simulink model "simTopLevel"  (R2016b)
settings: Solver=ode15s  StartTime=0.0  StopTime=2  RelTol=1e-3  EnableMultiTasking=on
InitFcn:
  | % minitaurParameters
model workspace (MAT data in the model file):
  MCOS : class17 (value not decoded)
  MCOS : class17 (value not decoded)
  MCOS : class17 (value not decoded)
  MCOS : class17 (value not decoded)
values from neighbouring files (symbols this model uses):
  controlParams = Simulink.Parameter(controlParams)    [minitaurParameters.m]
  envParams = Simulink.Parameter(envParams)    [minitaurParameters.m]
  IC = Simulink.Parameter(IC)    [minitaurParameters.m]
  minitaurParams = Simulink.Parameter(minitaurParams)    [minitaurParameters.m]
undefined symbols (not defined in the file or in its folder): Axis, Fn, ForeRearLag, Period, tau0, tau1, X, Y, Z
libraries: sm_lib x464, fl_lib x132, nesl_utility x41, Contact_Forces_Lib x28, simulink x13, simulink_extras x1
(part 11 of 13)

== system simTopLevel/GR Minitaur/minitaur_leg_linkages_III/Joint Friction Model1/Full ==
  Ideal Force Sensor : fl_lib/Mechanical/Mechanical Sensors/Ideal Force Sensor
  Ideal Translational Velocity Source : fl_lib/Mechanical/Mechanical Sources/Ideal Translational Velocity Source
  Joint Diameter : fl_lib/Physical Signals/Functions/PS Gain  gain=2*leg_joint_radius
  Joint Radius : fl_lib/Physical Signals/Functions/PS Gain  gain=leg_joint_radius
  Mechanical Translational Reference : fl_lib/Mechanical/Translational Elements/Mechanical Translational Reference
  Mechanical Translational Reference1 : fl_lib/Mechanical/Translational Elements/Mechanical Translational Reference
  PS Terminator : fl_lib/Physical Signals/Sinks/PS Terminator
  Translational Friction : fl_lib/Mechanical/Translational Elements/Translational Friction  brkwy_frc=mu_brk*Fn N  Col_frc=mu_k*Fn N  visc_coef=fric_visc_coeff N/(m/s)  trans_coef=trans_coeff s/m  vel_thr=linear_region_thresh m/s  v_specify=off  v_priority=None  v=0 m/s  f_specify=off  f_priority=None  f=0 N
  Joint Angular Velocity : PMIOPort  Port=1  Side=Left
  Joint Force : PMIOPort  Port=2  Side=Left
  Friction Torque : PMIOPort  Port=3  Side=Right
  connections:
  Mechanical Translational Reference/LConn1 -- Ideal Force Sensor/RConn1
  Translational Friction/LConn1 -- Ideal Force Sensor/LConn1
  Translational Friction/RConn1 -- Ideal Translational Velocity Source/LConn1
  Ideal Force Sensor/RConn2 -- Joint Diameter/LConn1
  Joint Diameter/RConn1 -- Friction Torque/RConn1
  Mechanical Translational Reference1/LConn1 -- Ideal Translational Velocity Source/RConn2
  Joint Force/RConn1 -- PS Terminator/LConn1
  Joint Radius/LConn1 -- Joint Angular Velocity/RConn1
  Joint Radius/RConn1 -- Ideal Translational Velocity Source/RConn1

== system simTopLevel/GR Minitaur/minitaur_leg_linkages_III/Joint Friction Model1/Stick-Slip ==
  Joint Diameter : fl_lib/Physical Signals/Functions/PS Gain  gain=2*leg_joint_radius
  Joint Radius : fl_lib/Physical Signals/Functions/PS Gain  gain=leg_joint_radius
  PS Add : fl_lib/Physical Signals/Functions/PS Add
  Stick-Slip Friction X : Contact_Forces_Lib/Friction Utilities/Stick-Slip Friction 1D  fn_axis=X-Axis  mu_kinetic=mu_k/2  mu_static=mu_s/2  vel_th=linear_region_thresh  filt_const=1/(2*pi*fric_bandwidth)
  Stick-Slip Friction Y : Contact_Forces_Lib/Friction Utilities/Stick-Slip Friction 1D  fn_axis=Y-Axis  mu_kinetic=mu_k/2  mu_static=mu_s/2  vel_th=linear_region_thresh  filt_const=1/(2*pi*fric_bandwidth)
  Joint Angular Velocity : PMIOPort  Port=1  Side=Left
  Joint Force : PMIOPort  Port=2  Side=Left
  Friction Torque : PMIOPort  Port=3  Side=Right
  connections:
  Joint Radius/RConn1 -- Stick-Slip Friction X/LConn2 -- Stick-Slip Friction Y/LConn2
  Joint Force/RConn1 -- Stick-Slip Friction X/LConn1 -- Stick-Slip Friction Y/LConn1
  Stick-Slip Friction Y/RConn1 -- PS Add/LConn2
  Stick-Slip Friction X/RConn1 -- PS Add/LConn1
  Joint Diameter/LConn1 -- PS Add/RConn1
  Joint Diameter/RConn1 -- Friction Torque/RConn1
  Joint Radius/LConn1 -- Joint Angular Velocity/RConn1

== system simTopLevel/GR Minitaur/minitaur_leg_linkages_III/Joint Friction Model2/Full ==
  Ideal Force Sensor : fl_lib/Mechanical/Mechanical Sensors/Ideal Force Sensor
  Ideal Translational Velocity Source : fl_lib/Mechanical/Mechanical Sources/Ideal Translational Velocity Source
  Joint Diameter : fl_lib/Physical Signals/Functions/PS Gain  gain=2*leg_joint_radius
  Joint Radius : fl_lib/Physical Signals/Functions/PS Gain  gain=leg_joint_radius
  Mechanical Translational Reference : fl_lib/Mechanical/Translational Elements/Mechanical Translational Reference
  Mechanical Translational Reference1 : fl_lib/Mechanical/Translational Elements/Mechanical Translational Reference
  PS Terminator : fl_lib/Physical Signals/Sinks/PS Terminator
  Translational Friction : fl_lib/Mechanical/Translational Elements/Translational Friction  brkwy_frc=mu_brk*Fn N  Col_frc=mu_k*Fn N  visc_coef=fric_visc_coeff N/(m/s)  trans_coef=trans_coeff s/m  vel_thr=linear_region_thresh m/s  v_specify=off  v_priority=None  v=0 m/s  f_specify=off  f_priority=None  f=0 N
  Joint Angular Velocity : PMIOPort  Port=1  Side=Left
  Joint Force : PMIOPort  Port=2  Side=Left
  Friction Torque : PMIOPort  Port=3  Side=Right
  connections:
  Mechanical Translational Reference/LConn1 -- Ideal Force Sensor/RConn1
  Translational Friction/LConn1 -- Ideal Force Sensor/LConn1
  Translational Friction/RConn1 -- Ideal Translational Velocity Source/LConn1
  Ideal Force Sensor/RConn2 -- Joint Diameter/LConn1
  Joint Diameter/RConn1 -- Friction Torque/RConn1
  Mechanical Translational Reference1/LConn1 -- Ideal Translational Velocity Source/RConn2
  Joint Force/RConn1 -- PS Terminator/LConn1
  Joint Radius/LConn1 -- Joint Angular Velocity/RConn1
  Joint Radius/RConn1 -- Ideal Translational Velocity Source/RConn1

== system simTopLevel/GR Minitaur/minitaur_leg_linkages_III/Joint Friction Model2/Stick-Slip ==
  Joint Diameter : fl_lib/Physical Signals/Functions/PS Gain  gain=2*leg_joint_radius
  Joint Radius : fl_lib/Physical Signals/Functions/PS Gain  gain=leg_joint_radius
  PS Add : fl_lib/Physical Signals/Functions/PS Add
  Stick-Slip Friction X : Contact_Forces_Lib/Friction Utilities/Stick-Slip Friction 1D  fn_axis=X-Axis  mu_kinetic=mu_k/2  mu_static=mu_s/2  vel_th=linear_region_thresh  filt_const=1/(2*pi*fric_bandwidth)
  Stick-Slip Friction Y : Contact_Forces_Lib/Friction Utilities/Stick-Slip Friction 1D  fn_axis=Y-Axis  mu_kinetic=mu_k/2  mu_static=mu_s/2  vel_th=linear_region_thresh  filt_const=1/(2*pi*fric_bandwidth)
  Joint Angular Velocity : PMIOPort  Port=1  Side=Left
  Joint Force : PMIOPort  Port=2  Side=Left
  Friction Torque : PMIOPort  Port=3  Side=Right
  connections:
  Joint Radius/RConn1 -- Stick-Slip Friction X/LConn2 -- Stick-Slip Friction Y/LConn2
  Joint Force/RConn1 -- Stick-Slip Friction X/LConn1 -- Stick-Slip Friction Y/LConn1
  Stick-Slip Friction Y/RConn1 -- PS Add/LConn2
  Stick-Slip Friction X/RConn1 -- PS Add/LConn1
  Joint Diameter/LConn1 -- PS Add/RConn1
  Joint Diameter/RConn1 -- Friction Torque/RConn1
  Joint Radius/LConn1 -- Joint Angular Velocity/RConn1

== system simTopLevel/GR Minitaur/minitaur_leg_linkages_IV/Joint Friction Model/Full ==
  Ideal Force Sensor : fl_lib/Mechanical/Mechanical Sensors/Ideal Force Sensor
  Ideal Translational Velocity Source : fl_lib/Mechanical/Mechanical Sources/Ideal Translational Velocity Source
  Joint Diameter : fl_lib/Physical Signals/Functions/PS Gain  gain=2*leg_joint_radius
  Joint Radius : fl_lib/Physical Signals/Functions/PS Gain  gain=leg_joint_radius
  Mechanical Translational Reference : fl_lib/Mechanical/Translational Elements/Mechanical Translational Reference
  Mechanical Translational Reference1 : fl_lib/Mechanical/Translational Elements/Mechanical Translational Reference
  PS Terminator : fl_lib/Physical Signals/Sinks/PS Terminator
  Translational Friction : fl_lib/Mechanical/Translational Elements/Translational Friction  brkwy_frc=mu_brk*Fn N  Col_frc=mu_k*Fn N  visc_coef=fric_visc_coeff N/(m/s)  trans_coef=trans_coeff s/m  vel_thr=linear_region_thresh m/s  v_specify=off  v_priority=None  v=0 m/s  f_specify=off  f_priority=None  f=0 N
  Joint Angular Velocity : PMIOPort  Port=1  Side=Left
  Joint Force : PMIOPort  Port=2  Side=Left
  Friction Torque : PMIOPort  Port=3  Side=Right
  connections:
  Mechanical Translational Reference/LConn1 -- Ideal Force Sensor/RConn1
  Translational Friction/LConn1 -- Ideal Force Sensor/LConn1
  Translational Friction/RConn1 -- Ideal Translational Velocity Source/LConn1
  Ideal Force Sensor/RConn2 -- Joint Diameter/LConn1
  Joint Diameter/RConn1 -- Friction Torque/RConn1
  Mechanical Translational Reference1/LConn1 -- Ideal Translational Velocity Source/RConn2
  Joint Force/RConn1 -- PS Terminator/LConn1
  Joint Radius/LConn1 -- Joint Angular Velocity/RConn1
  Joint Radius/RConn1 -- Ideal Translational Velocity Source/RConn1

== system simTopLevel/GR Minitaur/minitaur_leg_linkages_IV/Joint Friction Model/Stick-Slip ==
  Joint Diameter : fl_lib/Physical Signals/Functions/PS Gain  gain=2*leg_joint_radius
  Joint Radius : fl_lib/Physical Signals/Functions/PS Gain  gain=leg_joint_radius
  PS Add : fl_lib/Physical Signals/Functions/PS Add
  Stick-Slip Friction X : Contact_Forces_Lib/Friction Utilities/Stick-Slip Friction 1D  fn_axis=X-Axis  mu_kinetic=mu_k/2  mu_static=mu_s/2  vel_th=linear_region_thresh  filt_const=1/(2*pi*fric_bandwidth)
  Stick-Slip Friction Y : Contact_Forces_Lib/Friction Utilities/Stick-Slip Friction 1D  fn_axis=Y-Axis  mu_kinetic=mu_k/2  mu_static=mu_s/2  vel_th=linear_region_thresh  filt_const=1/(2*pi*fric_bandwidth)
  Joint Angular Velocity : PMIOPort  Port=1  Side=Left
  Joint Force : PMIOPort  Port=2  Side=Left
  Friction Torque : PMIOPort  Port=3  Side=Right
  connections:
  Joint Radius/RConn1 -- Stick-Slip Friction X/LConn2 -- Stick-Slip Friction Y/LConn2
  Joint Force/RConn1 -- Stick-Slip Friction X/LConn1 -- Stick-Slip Friction Y/LConn1
  Stick-Slip Friction Y/RConn1 -- PS Add/LConn2
  Stick-Slip Friction X/RConn1 -- PS Add/LConn1
  Joint Diameter/LConn1 -- PS Add/RConn1
  Joint Diameter/RConn1 -- Friction Torque/RConn1
  Joint Radius/LConn1 -- Joint Angular Velocity/RConn1

== system simTopLevel/GR Minitaur/minitaur_leg_linkages_IV/Joint Friction Model1/Full ==
  Ideal Force Sensor : fl_lib/Mechanical/Mechanical Sensors/Ideal Force Sensor
  Ideal Translational Velocity Source : fl_lib/Mechanical/Mechanical Sources/Ideal Translational Velocity Source
  Joint Diameter : fl_lib/Physical Signals/Functions/PS Gain  gain=2*leg_joint_radius
  Joint Radius : fl_lib/Physical Signals/Functions/PS Gain  gain=leg_joint_radius
  Mechanical Translational Reference : fl_lib/Mechanical/Translational Elements/Mechanical Translational Reference
  Mechanical Translational Reference1 : fl_lib/Mechanical/Translational Elements/Mechanical Translational Reference
  PS Terminator : fl_lib/Physical Signals/Sinks/PS Terminator
  Translational Friction : fl_lib/Mechanical/Translational Elements/Translational Friction  brkwy_frc=mu_brk*Fn N  Col_frc=mu_k*Fn N  visc_coef=fric_visc_coeff N/(m/s)  trans_coef=trans_coeff s/m  vel_thr=linear_region_thresh m/s  v_specify=off  v_priority=None  v=0 m/s  f_specify=off  f_priority=None  f=0 N
  Joint Angular Velocity : PMIOPort  Port=1  Side=Left
  Joint Force : PMIOPort  Port=2  Side=Left
  Friction Torque : PMIOPort  Port=3  Side=Right
  connections:
  Mechanical Translational Reference/LConn1 -- Ideal Force Sensor/RConn1
  Translational Friction/LConn1 -- Ideal Force Sensor/LConn1
  Translational Friction/RConn1 -- Ideal Translational Velocity Source/LConn1
  Ideal Force Sensor/RConn2 -- Joint Diameter/LConn1
  Joint Diameter/RConn1 -- Friction Torque/RConn1
  Mechanical Translational Reference1/LConn1 -- Ideal Translational Velocity Source/RConn2
  Joint Force/RConn1 -- PS Terminator/LConn1
  Joint Radius/LConn1 -- Joint Angular Velocity/RConn1
  Joint Radius/RConn1 -- Ideal Translational Velocity Source/RConn1

== system simTopLevel/GR Minitaur/minitaur_leg_linkages_IV/Joint Friction Model1/Stick-Slip ==
  Joint Diameter : fl_lib/Physical Signals/Functions/PS Gain  gain=2*leg_joint_radius
  Joint Radius : fl_lib/Physical Signals/Functions/PS Gain  gain=leg_joint_radius
  PS Add : fl_lib/Physical Signals/Functions/PS Add
  Stick-Slip Friction X : Contact_Forces_Lib/Friction Utilities/Stick-Slip Friction 1D  fn_axis=X-Axis  mu_kinetic=mu_k/2  mu_static=mu_s/2  vel_th=linear_region_thresh  filt_const=1/(2*pi*fric_bandwidth)
  Stick-Slip Friction Y : Contact_Forces_Lib/Friction Utilities/Stick-Slip Friction 1D  fn_axis=Y-Axis  mu_kinetic=mu_k/2  mu_static=mu_s/2  vel_th=linear_region_thresh  filt_const=1/(2*pi*fric_bandwidth)
  Joint Angular Velocity : PMIOPort  Port=1  Side=Left
  Joint Force : PMIOPort  Port=2  Side=Left
  Friction Torque : PMIOPort  Port=3  Side=Right
  connections:
  Joint Radius/RConn1 -- Stick-Slip Friction X/LConn2 -- Stick-Slip Friction Y/LConn2
  Joint Force/RConn1 -- Stick-Slip Friction X/LConn1 -- Stick-Slip Friction Y/LConn1
  Stick-Slip Friction Y/RConn1 -- PS Add/LConn2
  Stick-Slip Friction X/RConn1 -- PS Add/LConn1
  Joint Diameter/LConn1 -- PS Add/RConn1
  Joint Diameter/RConn1 -- Friction Torque/RConn1
  Joint Radius/LConn1 -- Joint Angular Velocity/RConn1

== system simTopLevel/GR Minitaur/minitaur_leg_linkages_IV/Joint Friction Model2/Full ==
  Ideal Force Sensor : fl_lib/Mechanical/Mechanical Sensors/Ideal Force Sensor
  Ideal Translational Velocity Source : fl_lib/Mechanical/Mechanical Sources/Ideal Translational Velocity Source
  Joint Diameter : fl_lib/Physical Signals/Functions/PS Gain  gain=2*leg_joint_radius
  Joint Radius : fl_lib/Physical Signals/Functions/PS Gain  gain=leg_joint_radius
  Mechanical Translational Reference : fl_lib/Mechanical/Translational Elements/Mechanical Translational Reference
  Mechanical Translational Reference1 : fl_lib/Mechanical/Translational Elements/Mechanical Translational Reference
  PS Terminator : fl_lib/Physical Signals/Sinks/PS Terminator
  Translational Friction : fl_lib/Mechanical/Translational Elements/Translational Friction  brkwy_frc=mu_brk*Fn N  Col_frc=mu_k*Fn N  visc_coef=fric_visc_coeff N/(m/s)  trans_coef=trans_coeff s/m  vel_thr=linear_region_thresh m/s  v_specify=off  v_priority=None  v=0 m/s  f_specify=off  f_priority=None  f=0 N
  Joint Angular Velocity : PMIOPort  Port=1  Side=Left
  Joint Force : PMIOPort  Port=2  Side=Left
  Friction Torque : PMIOPort  Port=3  Side=Right
  connections:
  Mechanical Translational Reference/LConn1 -- Ideal Force Sensor/RConn1
  Translational Friction/LConn1 -- Ideal Force Sensor/LConn1
  Translational Friction/RConn1 -- Ideal Translational Velocity Source/LConn1
  Ideal Force Sensor/RConn2 -- Joint Diameter/LConn1
  Joint Diameter/RConn1 -- Friction Torque/RConn1
  Mechanical Translational Reference1/LConn1 -- Ideal Translational Velocity Source/RConn2
  Joint Force/RConn1 -- PS Terminator/LConn1
  Joint Radius/LConn1 -- Joint Angular Velocity/RConn1
  Joint Radius/RConn1 -- Ideal Translational Velocity Source/RConn1

== system simTopLevel/GR Minitaur/minitaur_leg_linkages_IV/Joint Friction Model2/Stick-Slip ==
  Joint Diameter : fl_lib/Physical Signals/Functions/PS Gain  gain=2*leg_joint_radius
  Joint Radius : fl_lib/Physical Signals/Functions/PS Gain  gain=leg_joint_radius
  PS Add : fl_lib/Physical Signals/Functions/PS Add
  Stick-Slip Friction X : Contact_Forces_Lib/Friction Utilities/Stick-Slip Friction 1D  fn_axis=X-Axis  mu_kinetic=mu_k/2  mu_static=mu_s/2  vel_th=linear_region_thresh  filt_const=1/(2*pi*fric_bandwidth)
  Stick-Slip Friction Y : Contact_Forces_Lib/Friction Utilities/Stick-Slip Friction 1D  fn_axis=Y-Axis  mu_kinetic=mu_k/2  mu_static=mu_s/2  vel_th=linear_region_thresh  filt_const=1/(2*pi*fric_bandwidth)
  Joint Angular Velocity : PMIOPort  Port=1  Side=Left
  Joint Force : PMIOPort  Port=2  Side=Left
  Friction Torque : PMIOPort  Port=3  Side=Right
  connections:
  Joint Radius/RConn1 -- Stick-Slip Friction X/LConn2 -- Stick-Slip Friction Y/LConn2
  Joint Force/RConn1 -- Stick-Slip Friction X/LConn1 -- Stick-Slip Friction Y/LConn1
  Stick-Slip Friction Y/RConn1 -- PS Add/LConn2
  Stick-Slip Friction X/RConn1 -- PS Add/LConn1
  Joint Diameter/LConn1 -- PS Add/RConn1
  Joint Diameter/RConn1 -- Friction Torque/RConn1
  Joint Radius/LConn1 -- Joint Angular Velocity/RConn1

== system simTopLevel/GR Minitaur/minitaur_motor_module_IA/DYS_BLDC_86x10_BE8108_12/BLDC Model ==
  Desired Torque  [Nm] : Inport
  Velocity [rad/s] : Inport  Port=2
  Constant : Constant  Value=torque_sat
  Constant1 : Constant  Value=-torque_sat
  Gain : Gain  Gain=1/kt
  Gain1 : Gain  Gain=r
  Math Function : Math  Operator=square  SaturateOnIntegerOverflow=on
  Saturation Dynamic : simulink/Discontinuities/Saturation Dynamic  OutMin=[]  OutMax=[]  OutDataTypeStr=Inherit: Same as second input  OutDataType=fixdt(1, 16)  OutScaling=2^-10  DoSatur=off
  Terminator : Terminator
  Transfer Fcn : TransferFcn  Denominator=[timeconst 1]
  Torque [N*m] : Outport
  Ploss [W] : Outport  Port=2
  wires:
  Desired Torque  [Nm]/1 -> Transfer Fcn/1
  Math Function/1 -> Gain1/1
  Gain/1 -> Math Function/1
  Gain1/1 -> Ploss [W]/1
  Velocity [rad/s]/1 -> Terminator/1
  Transfer Fcn/1 -> Saturation Dynamic/2
  Saturation Dynamic/1 -> Gain/1, Torque [N*m]/1
  Constant/1 -> Saturation Dynamic/1
  Constant1/1 -> Saturation Dynamic/3

== system simTopLevel/GR Minitaur/minitaur_motor_module_IA/DYS_BLDC_86x10_BE8108_12/DYS_BLDC_86x10_BE8108_12_rotor_1_RIGID ==
  ReferenceFrame : sm_lib/Frames and Transforms/Reference Frame
  Solid : sm_lib/Body Elements/Solid  InertiaType=Custom  Mass=minitaurParams.Solid(7).mass  MassUnits=kg  CenterOfMass=minitaurParams.Solid(7).CoM  CenterOfMassUnits=mm  MomentsOfInertia=minitaurParams.Solid(7).MoI  MomentsOfInertiaUnits=kg*mm^2  ProductsOfInertia=minitaurParams.Solid(7).PoI  ProductsOfInertiaUnits=kg*mm^2  DensityBased=on  Density=1000  DensityUnits=kg/(m^3)  DoExposeReferenceFrame=on  SerializedFrames=<Frames/>  GraphicType=FromGeometry  MarkerShape=Sphere  MarkerSize=10  GraphicVisPropType=SimpleVisualProperties  GraphicDiffuseColor=minitaurParams.Solid(7).color  GraphicSpecularColor=[0.5 0.5 0.5 1.0]  GraphicAmbientColor=[0.15 0.15 0.15 1.0]  GraphicEmissiveColor=[0.0 0.0 0.0 1.0]  GraphicShininess=75  GraphicOpacity=minitaurParams.Solid(7).opacity  GeometryShape=FromFile  RectangleSize=[1 1]  RectangleSizeUnits=m  BrickDimensions=[1 1 1]  BrickDimensionUnits=m  CylinderRadius=1  CylinderRadiusUnits=m  CylinderLength=1  CylinderLengthUnits=m  SphereRadius=1  SphereRadiusUnits=m  EllipsoidRadii=[1 1 1]  EllipsoidRadiiUnits=m  ExtrusionCrossSection=[1 1; -1 1; -1 -1; 1 -1]  ExtrusionCrossSectionUnits=m  ExtrusionLength=1  ExtrusionLengthUnits=m  PolygonNumSides=3  PolygonOuterRadius=1  PolygonOuterRadiusUnits=m  ExtGeomFileType=STEP  ExtGeomFileName=model/DYS-BLDC-86x10-BE8108-12-rotor_Default_sldprt.STEP  ExtGeomFileUnits=m  RevolutionCrossSection=[1 1; 1 -1; 2 -1; 2 1]  RevolutionCrossSectionUnits=m  RevolutionExtent=Full  RevolutionAngle=180  RevolutionAngleUnits=deg
  Transform : sm_lib/Frames and Transforms/Rigid Transform  TranslationMethod=Cartesian  TranslationStandardOffset=0  TranslationLengthUnit=mm  TranslationStandardAxis=+Z  TranslationCartesianOffset=minitaurParams.RigidTransform(20).translation  TranslationROffset=0  TranslationROffsetUnits=m  TranslationZOffset=0  TranslationZOffsetUnits=m  TranslationThetaOffset=0  TranslationThetaOffsetUnits=deg  RotationMethod=ArbitraryAxis  RotationAngleUnits=rad  RotationStandardAxis=+Z  RotationAngle=minitaurParams.RigidTransform(20).angle  RotationArbitraryAxis=minitaurParams.RigidTransform(20).axis  FollAlignAxisA=+X  BaseAlignAxisA=+Y  FollAlignAxisB=+Y  BaseAlignAxisB=+Z  RotationSequenceAxes=FollowerAxes  RotationSequence=XYX  RotationSequenceAngles=[0 0 0]  RotationSequenceAnglesUnits=deg  RotationMatrix=[1 0 0; 0 1 0; 0 0 1]
  Transform1 : sm_lib/Frames and Transforms/Rigid Transform  TranslationMethod=Cartesian  TranslationStandardOffset=0  TranslationLengthUnit=mm  TranslationStandardAxis=+Z  TranslationCartesianOffset=minitaurParams.RigidTransform(48).translation  TranslationROffset=0  TranslationROffsetUnits=m  TranslationZOffset=0  TranslationZOffsetUnits=m  TranslationThetaOffset=0  TranslationThetaOffsetUnits=deg  RotationMethod=ArbitraryAxis  RotationAngleUnits=rad  RotationStandardAxis=+Z  RotationAngle=minitaurParams.RigidTransform(48).angle  RotationArbitraryAxis=minitaurParams.RigidTransform(48).axis  FollAlignAxisA=+X  BaseAlignAxisA=+Y  FollAlignAxisB=+Y  BaseAlignAxisB=+Z  RotationSequenceAxes=FollowerAxes  RotationSequence=XYX  RotationSequenceAngles=[0 0 0]  RotationSequenceAnglesUnits=deg  RotationMatrix=[1 0 0; 0 1 0; 0 0 1]
  F1 : PMIOPort  Port=1  Side=Left
  F : PMIOPort  Port=2  Side=Left
  connections:
  ReferenceFrame/RConn1 -- Solid/RConn1 -- Transform/LConn1 -- Transform1/LConn1
  Transform/RConn1 -- F/RConn1
  Transform1/RConn1 -- F1/RConn1

== system simTopLevel/GR Minitaur/minitaur_motor_module_IA/DYS_BLDC_86x10_BE8108_12/DYS_BLDC_86x10_BE8108_12_stator_1_RIGID ==
  ReferenceFrame : sm_lib/Frames and Transforms/Reference Frame
  Solid : sm_lib/Body Elements/Solid  InertiaType=Custom  Mass=minitaurParams.Solid(6).mass  MassUnits=kg  CenterOfMass=minitaurParams.Solid(6).CoM  CenterOfMassUnits=mm  MomentsOfInertia=minitaurParams.Solid(6).MoI  MomentsOfInertiaUnits=kg*mm^2  ProductsOfInertia=minitaurParams.Solid(6).PoI  ProductsOfInertiaUnits=kg*mm^2  DensityBased=on  Density=1000  DensityUnits=kg/(m^3)  DoExposeReferenceFrame=on  SerializedFrames=<Frames/>  GraphicType=FromGeometry  MarkerShape=Sphere  MarkerSize=10  GraphicVisPropType=SimpleVisualProperties  GraphicDiffuseColor=minitaurParams.Solid(6).color  GraphicSpecularColor=[0.5 0.5 0.5 1.0]  GraphicAmbientColor=[0.15 0.15 0.15 1.0]  GraphicEmissiveColor=[0.0 0.0 0.0 1.0]  GraphicShininess=75  GraphicOpacity=minitaurParams.Solid(6).opacity  GeometryShape=FromFile  RectangleSize=[1 1]  RectangleSizeUnits=m  BrickDimensions=[1 1 1]  BrickDimensionUnits=m  CylinderRadius=1  CylinderRadiusUnits=m  CylinderLength=1  CylinderLengthUnits=m  SphereRadius=1  SphereRadiusUnits=m  EllipsoidRadii=[1 1 1]  EllipsoidRadiiUnits=m  ExtrusionCrossSection=[1 1; -1 1; -1 -1; 1 -1]  ExtrusionCrossSectionUnits=m  ExtrusionLength=1  ExtrusionLengthUnits=m  PolygonNumSides=3  PolygonOuterRadius=1  PolygonOuterRadiusUnits=m  ExtGeomFileType=STEP  ExtGeomFileName=model/DYS-BLDC-86x10-BE8108-12-stator_Default_sldprt.STEP  ExtGeomFileUnits=m  RevolutionCrossSection=[1 1; 1 -1; 2 -1; 2 1]  RevolutionCrossSectionUnits=m  RevolutionExtent=Full  RevolutionAngle=180  RevolutionAngleUnits=deg
  Transform : sm_lib/Frames and Transforms/Rigid Transform  TranslationMethod=Cartesian  TranslationStandardOffset=0  TranslationLengthUnit=mm  TranslationStandardAxis=+Z  TranslationCartesianOffset=minitaurParams.RigidTransform(17).translation  TranslationROffset=0  TranslationROffsetUnits=m  TranslationZOffset=0  TranslationZOffsetUnits=m  TranslationThetaOffset=0  TranslationThetaOffsetUnits=deg  RotationMethod=ArbitraryAxis  RotationAngleUnits=rad  RotationStandardAxis=+Z  RotationAngle=minitaurParams.RigidTransform(17).angle  RotationArbitraryAxis=minitaurParams.RigidTransform(17).axis  FollAlignAxisA=+X  BaseAlignAxisA=+Y  FollAlignAxisB=+Y  BaseAlignAxisB=+Z  RotationSequenceAxes=FollowerAxes  RotationSequence=XYX  RotationSequenceAngles=[0 0 0]  RotationSequenceAnglesUnits=deg  RotationMatrix=[1 0 0; 0 1 0; 0 0 1]
  Transform1 : sm_lib/Frames and Transforms/Rigid Transform  TranslationMethod=Cartesian  TranslationStandardOffset=0  TranslationLengthUnit=mm  TranslationStandardAxis=+Z  TranslationCartesianOffset=minitaurParams.RigidTransform(19).translation  TranslationROffset=0  TranslationROffsetUnits=m  TranslationZOffset=0  TranslationZOffsetUnits=m  TranslationThetaOffset=0  TranslationThetaOffsetUnits=deg  RotationMethod=ArbitraryAxis  RotationAngleUnits=rad  RotationStandardAxis=+Z  RotationAngle=minitaurParams.RigidTransform(19).angle  RotationArbitraryAxis=minitaurParams.RigidTransform(19).axis  FollAlignAxisA=+X  BaseAlignAxisA=+Y  FollAlignAxisB=+Y  BaseAlignAxisB=+Z  RotationSequenceAxes=FollowerAxes  RotationSequence=XYX  RotationSequenceAngles=[0 0 0]  RotationSequenceAnglesUnits=deg  RotationMatrix=[1 0 0; 0 1 0; 0 0 1]
  Transform2 : sm_lib/Frames and Transforms/Rigid Transform  TranslationMethod=Cartesian  TranslationStandardOffset=0  TranslationLengthUnit=mm  TranslationStandardAxis=+Z  TranslationCartesianOffset=minitaurParams.RigidTransform(26).translation  TranslationROffset=0  TranslationROffsetUnits=m  TranslationZOffset=0  TranslationZOffsetUnits=m  TranslationThetaOffset=0  TranslationThetaOffsetUnits=deg  RotationMethod=ArbitraryAxis  RotationAngleUnits=rad  RotationStandardAxis=+Z  RotationAngle=minitaurParams.RigidTransform(26).angle  RotationArbitraryAxis=minitaurParams.RigidTransform(26).axis  FollAlignAxisA=+X  BaseAlignAxisA=+Y  FollAlignAxisB=+Y  BaseAlignAxisB=+Z  RotationSequenceAxes=FollowerAxes  RotationSequence=XYX  RotationSequenceAngles=[0 0 0]  RotationSequenceAnglesUnits=deg  RotationMatrix=[1 0 0; 0 1 0; 0 0 1]
  Transform3 : sm_lib/Frames and Transforms/Rigid Transform  TranslationMethod=Cartesian  TranslationStandardOffset=0  TranslationLengthUnit=mm  TranslationStandardAxis=+Z  TranslationCartesianOffset=minitaurParams.RigidTransform(34).translation  TranslationROffset=0  TranslationROffsetUnits=m  TranslationZOffset=0  TranslationZOffsetUnits=m  TranslationThetaOffset=0  TranslationThetaOffsetUnits=deg  RotationMethod=ArbitraryAxis  RotationAngleUnits=rad  RotationStandardAxis=+Z  RotationAngle=minitaurParams.RigidTransform(34).angle  RotationArbitraryAxis=minitaurParams.RigidTransform(34).axis  FollAlignAxisA=+X  BaseAlignAxisA=+Y  FollAlignAxisB=+Y  BaseAlignAxisB=+Z  RotationSequenceAxes=FollowerAxes  RotationSequence=XYX  RotationSequenceAngles=[0 0 0]  RotationSequenceAnglesUnits=deg  RotationMatrix=[1 0 0; 0 1 0; 0 0 1]
  F2 : PMIOPort  Port=1  Side=Left
  F3 : PMIOPort  Port=2  Side=Left
  F : PMIOPort  Port=3  Side=Left
  F1 : PMIOPort  Port=4  Side=Right
  connections:
  Transform2/LConn1 -- Transform3/LConn1 -- ReferenceFrame/RConn1 -- Solid/RConn1 -- Transform/LConn1 -- Transform1/LConn1
  Transform/RConn1 -- F/RConn1
  Transform1/RConn1 -- F1/RConn1
  Transform2/RConn1 -- F2/RConn1
  Transform3/RConn1 -- F3/RConn1

== system simTopLevel/GR Minitaur/minitaur_motor_module_IB/DYS_BLDC_86x10_BE8108_12/BLDC Model ==
  Desired Torque  [Nm] : Inport
  Velocity [rad/s] : Inport  Port=2
  Constant : Constant  Value=torque_sat
  Constant1 : Constant  Value=-torque_sat
  Gain : Gain  Gain=1/kt
  Gain1 : Gain  Gain=r
  Math Function : Math  Operator=square  SaturateOnIntegerOverflow=on
  Saturation Dynamic : simulink/Discontinuities/Saturation Dynamic  OutMin=[]  OutMax=[]  OutDataTypeStr=Inherit: Same as second input  OutDataType=fixdt(1, 16)  OutScaling=2^-10  DoSatur=off
  Terminator : Terminator
  Transfer Fcn : TransferFcn  Denominator=[timeconst 1]
  Torque [N*m] : Outport
  Ploss [W] : Outport  Port=2
  wires:
  Desired Torque  [Nm]/1 -> Transfer Fcn/1
  Math Function/1 -> Gain1/1
  Gain/1 -> Math Function/1
  Gain1/1 -> Ploss [W]/1
  Velocity [rad/s]/1 -> Terminator/1
  Transfer Fcn/1 -> Saturation Dynamic/2
  Saturation Dynamic/1 -> Gain/1, Torque [N*m]/1
  Constant/1 -> Saturation Dynamic/1
  Constant1/1 -> Saturation Dynamic/3

== system simTopLevel/GR Minitaur/minitaur_motor_module_IB/DYS_BLDC_86x10_BE8108_12/DYS_BLDC_86x10_BE8108_12_rotor_1_RIGID ==
  ReferenceFrame : sm_lib/Frames and Transforms/Reference Frame
  Solid : sm_lib/Body Elements/Solid  InertiaType=Custom  Mass=minitaurParams.Solid(7).mass  MassUnits=kg  CenterOfMass=minitaurParams.Solid(7).CoM  CenterOfMassUnits=mm  MomentsOfInertia=minitaurParams.Solid(7).MoI  MomentsOfInertiaUnits=kg*mm^2  ProductsOfInertia=minitaurParams.Solid(7).PoI  ProductsOfInertiaUnits=kg*mm^2  DensityBased=on  Density=1000  DensityUnits=kg/(m^3)  DoExposeReferenceFrame=on  SerializedFrames=<Frames/>  GraphicType=FromGeometry  MarkerShape=Sphere  MarkerSize=10  GraphicVisPropType=SimpleVisualProperties  GraphicDiffuseColor=minitaurParams.Solid(7).color  GraphicSpecularColor=[0.5 0.5 0.5 1.0]  GraphicAmbientColor=[0.15 0.15 0.15 1.0]  GraphicEmissiveColor=[0.0 0.0 0.0 1.0]  GraphicShininess=75  GraphicOpacity=minitaurParams.Solid(7).opacity  GeometryShape=FromFile  RectangleSize=[1 1]  RectangleSizeUnits=m  BrickDimensions=[1 1 1]  BrickDimensionUnits=m  CylinderRadius=1  CylinderRadiusUnits=m  CylinderLength=1  CylinderLengthUnits=m  SphereRadius=1  SphereRadiusUnits=m  EllipsoidRadii=[1 1 1]  EllipsoidRadiiUnits=m  ExtrusionCrossSection=[1 1; -1 1; -1 -1; 1 -1]  ExtrusionCrossSectionUnits=m  ExtrusionLength=1  ExtrusionLengthUnits=m  PolygonNumSides=3  PolygonOuterRadius=1  PolygonOuterRadiusUnits=m  ExtGeomFileType=STEP  ExtGeomFileName=model/DYS-BLDC-86x10-BE8108-12-rotor_Default_sldprt.STEP  ExtGeomFileUnits=m  RevolutionCrossSection=[1 1; 1 -1; 2 -1; 2 1]  RevolutionCrossSectionUnits=m  RevolutionExtent=Full  RevolutionAngle=180  RevolutionAngleUnits=deg
  Transform : sm_lib/Frames and Transforms/Rigid Transform  TranslationMethod=Cartesian  TranslationStandardOffset=0  TranslationLengthUnit=mm  TranslationStandardAxis=+Z  TranslationCartesianOffset=minitaurParams.RigidTransform(20).translation  TranslationROffset=0  TranslationROffsetUnits=m  TranslationZOffset=0  TranslationZOffsetUnits=m  TranslationThetaOffset=0  TranslationThetaOffsetUnits=deg  RotationMethod=ArbitraryAxis  RotationAngleUnits=rad  RotationStandardAxis=+Z  RotationAngle=minitaurParams.RigidTransform(20).angle  RotationArbitraryAxis=minitaurParams.RigidTransform(20).axis  FollAlignAxisA=+X  BaseAlignAxisA=+Y  FollAlignAxisB=+Y  BaseAlignAxisB=+Z  RotationSequenceAxes=FollowerAxes  RotationSequence=XYX  RotationSequenceAngles=[0 0 0]  RotationSequenceAnglesUnits=deg  RotationMatrix=[1 0 0; 0 1 0; 0 0 1]
  Transform1 : sm_lib/Frames and Transforms/Rigid Transform  TranslationMethod=Cartesian  TranslationStandardOffset=0  TranslationLengthUnit=mm  TranslationStandardAxis=+Z  TranslationCartesianOffset=minitaurParams.RigidTransform(50).translation  TranslationROffset=0  TranslationROffsetUnits=m  TranslationZOffset=0  TranslationZOffsetUnits=m  TranslationThetaOffset=0  TranslationThetaOffsetUnits=deg  RotationMethod=ArbitraryAxis  RotationAngleUnits=rad  RotationStandardAxis=+Z  RotationAngle=minitaurParams.RigidTransform(50).angle  RotationArbitraryAxis=minitaurParams.RigidTransform(50).axis  FollAlignAxisA=+X  BaseAlignAxisA=+Y  FollAlignAxisB=+Y  BaseAlignAxisB=+Z  RotationSequenceAxes=FollowerAxes  RotationSequence=XYX  RotationSequenceAngles=[0 0 0]  RotationSequenceAnglesUnits=deg  RotationMatrix=[1 0 0; 0 1 0; 0 0 1]
  F1 : PMIOPort  Port=1  Side=Left
  F : PMIOPort  Port=2  Side=Left
  connections:
  ReferenceFrame/RConn1 -- Transform/LConn1 -- Transform1/LConn1 -- Solid/RConn1
  Transform/RConn1 -- F/RConn1
  Transform1/RConn1 -- F1/RConn1

== system simTopLevel/GR Minitaur/minitaur_motor_module_IB/DYS_BLDC_86x10_BE8108_12/DYS_BLDC_86x10_BE8108_12_stator_1_RIGID ==
  ReferenceFrame : sm_lib/Frames and Transforms/Reference Frame
  Solid : sm_lib/Body Elements/Solid  InertiaType=Custom  Mass=minitaurParams.Solid(6).mass  MassUnits=kg  CenterOfMass=minitaurParams.Solid(6).CoM  CenterOfMassUnits=mm  MomentsOfInertia=minitaurParams.Solid(6).MoI  MomentsOfInertiaUnits=kg*mm^2  ProductsOfInertia=minitaurParams.Solid(6).PoI  ProductsOfInertiaUnits=kg*mm^2  DensityBased=on  Density=1000  DensityUnits=kg/(m^3)  DoExposeReferenceFrame=on  SerializedFrames=<Frames/>  GraphicType=FromGeometry  MarkerShape=Sphere  MarkerSize=10  GraphicVisPropType=SimpleVisualProperties  GraphicDiffuseColor=minitaurParams.Solid(6).color  GraphicSpecularColor=[0.5 0.5 0.5 1.0]  GraphicAmbientColor=[0.15 0.15 0.15 1.0]  GraphicEmissiveColor=[0.0 0.0 0.0 1.0]  GraphicShininess=75  GraphicOpacity=minitaurParams.Solid(6).opacity  GeometryShape=FromFile  RectangleSize=[1 1]  RectangleSizeUnits=m  BrickDimensions=[1 1 1]  BrickDimensionUnits=m  CylinderRadius=1  CylinderRadiusUnits=m  CylinderLength=1  CylinderLengthUnits=m  SphereRadius=1  SphereRadiusUnits=m  EllipsoidRadii=[1 1 1]  EllipsoidRadiiUnits=m  ExtrusionCrossSection=[1 1; -1 1; -1 -1; 1 -1]  ExtrusionCrossSectionUnits=m  ExtrusionLength=1  ExtrusionLengthUnits=m  PolygonNumSides=3  PolygonOuterRadius=1  PolygonOuterRadiusUnits=m  ExtGeomFileType=STEP  ExtGeomFileName=model/DYS-BLDC-86x10-BE8108-12-stator_Default_sldprt.STEP  ExtGeomFileUnits=m  RevolutionCrossSection=[1 1; 1 -1; 2 -1; 2 1]  RevolutionCrossSectionUnits=m  RevolutionExtent=Full  RevolutionAngle=180  RevolutionAngleUnits=deg
  Transform : sm_lib/Frames and Transforms/Rigid Transform  TranslationMethod=Cartesian  TranslationStandardOffset=0  TranslationLengthUnit=mm  TranslationStandardAxis=+Z  TranslationCartesianOffset=minitaurParams.RigidTransform(17).translation  TranslationROffset=0  TranslationROffsetUnits=m  TranslationZOffset=0  TranslationZOffsetUnits=m  TranslationThetaOffset=0  TranslationThetaOffsetUnits=deg  RotationMethod=ArbitraryAxis  RotationAngleUnits=rad  RotationStandardAxis=+Z  RotationAngle=minitaurParams.RigidTransform(17).angle  RotationArbitraryAxis=minitaurParams.RigidTransform(17).axis  FollAlignAxisA=+X  BaseAlignAxisA=+Y  FollAlignAxisB=+Y  BaseAlignAxisB=+Z  RotationSequenceAxes=FollowerAxes  RotationSequence=XYX  RotationSequenceAngles=[0 0 0]  RotationSequenceAnglesUnits=deg  RotationMatrix=[1 0 0; 0 1 0; 0 0 1]
  Transform1 : sm_lib/Frames and Transforms/Rigid Transform  TranslationMethod=Cartesian  TranslationStandardOffset=0  TranslationLengthUnit=mm  TranslationStandardAxis=+Z  TranslationCartesianOffset=minitaurParams.RigidTransform(19).translation  TranslationROffset=0  TranslationROffsetUnits=m  TranslationZOffset=0  TranslationZOffsetUnits=m  TranslationThetaOffset=0  TranslationThetaOffsetUnits=deg  RotationMethod=ArbitraryAxis  RotationAngleUnits=rad  RotationStandardAxis=+Z  RotationAngle=minitaurParams.RigidTransform(19).angle  RotationArbitraryAxis=minitaurParams.RigidTransform(19).axis  FollAlignAxisA=+X  BaseAlignAxisA=+Y  FollAlignAxisB=+Y  BaseAlignAxisB=+Z  RotationSequenceAxes=FollowerAxes  RotationSequence=XYX  RotationSequenceAngles=[0 0 0]  RotationSequenceAnglesUnits=deg  RotationMatrix=[1 0 0; 0 1 0; 0 0 1]
  Transform2 : sm_lib/Frames and Transforms/Rigid Transform  TranslationMethod=Cartesian  TranslationStandardOffset=0  TranslationLengthUnit=mm  TranslationStandardAxis=+Z  TranslationCartesianOffset=minitaurParams.RigidTransform(26).translation  TranslationROffset=0  TranslationROffsetUnits=m  TranslationZOffset=0  TranslationZOffsetUnits=m  TranslationThetaOffset=0  TranslationThetaOffsetUnits=deg  RotationMethod=ArbitraryAxis  RotationAngleUnits=rad  RotationStandardAxis=+Z  RotationAngle=minitaurParams.RigidTransform(26).angle  RotationArbitraryAxis=minitaurParams.RigidTransform(26).axis  FollAlignAxisA=+X  BaseAlignAxisA=+Y  FollAlignAxisB=+Y  BaseAlignAxisB=+Z  RotationSequenceAxes=FollowerAxes  RotationSequence=XYX  RotationSequenceAngles=[0 0 0]  RotationSequenceAnglesUnits=deg  RotationMatrix=[1 0 0; 0 1 0; 0 0 1]
  Transform3 : sm_lib/Frames and Transforms/Rigid Transform  TranslationMethod=Cartesian  TranslationStandardOffset=0  TranslationLengthUnit=mm  TranslationStandardAxis=+Z  TranslationCartesianOffset=minitaurParams.RigidTransform(42).translation  TranslationROffset=0  TranslationROffsetUnits=m  TranslationZOffset=0  TranslationZOffsetUnits=m  TranslationThetaOffset=0  TranslationThetaOffsetUnits=deg  RotationMethod=ArbitraryAxis  RotationAngleUnits=rad  RotationStandardAxis=+Z  RotationAngle=minitaurParams.RigidTransform(42).angle  RotationArbitraryAxis=minitaurParams.RigidTransform(42).axis  FollAlignAxisA=+X  BaseAlignAxisA=+Y  FollAlignAxisB=+Y  BaseAlignAxisB=+Z  RotationSequenceAxes=FollowerAxes  RotationSequence=XYX  RotationSequenceAngles=[0 0 0]  RotationSequenceAnglesUnits=deg  RotationMatrix=[1 0 0; 0 1 0; 0 0 1]
  F2 : PMIOPort  Port=1  Side=Left
  F3 : PMIOPort  Port=2  Side=Left
  F : PMIOPort  Port=3  Side=Left
  F1 : PMIOPort  Port=4  Side=Right
  connections:
  ReferenceFrame/RConn1 -- Solid/RConn1 -- Transform/LConn1 -- Transform1/LConn1 -- Transform2/LConn1 -- Transform3/LConn1
  Transform/RConn1 -- F/RConn1
  Transform1/RConn1 -- F1/RConn1
  Transform2/RConn1 -- F2/RConn1
  Transform3/RConn1 -- F3/RConn1

== system simTopLevel/GR Minitaur/minitaur_motor_module_IIA/DYS_BLDC_86x10_BE8108_12/BLDC Model ==
  Desired Torque  [Nm] : Inport
  Velocity [rad/s] : Inport  Port=2
  Constant : Constant  Value=torque_sat
  Constant1 : Constant  Value=-torque_sat
  Gain : Gain  Gain=1/kt
  Gain1 : Gain  Gain=r
  Math Function : Math  Operator=square  SaturateOnIntegerOverflow=on
  Saturation Dynamic : simulink/Discontinuities/Saturation Dynamic  OutMin=[]  OutMax=[]  OutDataTypeStr=Inherit: Same as second input  OutDataType=fixdt(1, 16)  OutScaling=2^-10  DoSatur=off
  Terminator : Terminator
  Transfer Fcn : TransferFcn  Denominator=[timeconst 1]
  Torque [N*m] : Outport
  Ploss [W] : Outport  Port=2
  wires:
  Desired Torque  [Nm]/1 -> Transfer Fcn/1
  Math Function/1 -> Gain1/1
  Gain/1 -> Math Function/1
  Gain1/1 -> Ploss [W]/1
  Velocity [rad/s]/1 -> Terminator/1
  Transfer Fcn/1 -> Saturation Dynamic/2
  Saturation Dynamic/1 -> Gain/1, Torque [N*m]/1
  Constant/1 -> Saturation Dynamic/1
  Constant1/1 -> Saturation Dynamic/3

== system simTopLevel/GR Minitaur/minitaur_motor_module_IIA/DYS_BLDC_86x10_BE8108_12/DYS_BLDC_86x10_BE8108_12_rotor_1_RIGID ==
  ReferenceFrame : sm_lib/Frames and Transforms/Reference Frame
  Solid : sm_lib/Body Elements/Solid  InertiaType=Custom  Mass=minitaurParams.Solid(7).mass  MassUnits=kg  CenterOfMass=minitaurParams.Solid(7).CoM  CenterOfMassUnits=mm  MomentsOfInertia=minitaurParams.Solid(7).MoI  MomentsOfInertiaUnits=kg*mm^2  ProductsOfInertia=minitaurParams.Solid(7).PoI  ProductsOfInertiaUnits=kg*mm^2  DensityBased=on  Density=1000  DensityUnits=kg/(m^3)  DoExposeReferenceFrame=on  SerializedFrames=<Frames/>  GraphicType=FromGeometry  MarkerShape=Sphere  MarkerSize=10  GraphicVisPropType=SimpleVisualProperties  GraphicDiffuseColor=minitaurParams.Solid(7).color  GraphicSpecularColor=[0.5 0.5 0.5 1.0]  GraphicAmbientColor=[0.15 0.15 0.15 1.0]  GraphicEmissiveColor=[0.0 0.0 0.0 1.0]  GraphicShininess=75  GraphicOpacity=minitaurParams.Solid(7).opacity  GeometryShape=FromFile  RectangleSize=[1 1]  RectangleSizeUnits=m  BrickDimensions=[1 1 1]  BrickDimensionUnits=m  CylinderRadius=1  CylinderRadiusUnits=m  CylinderLength=1  CylinderLengthUnits=m  SphereRadius=1  SphereRadiusUnits=m  EllipsoidRadii=[1 1 1]  EllipsoidRadiiUnits=m  ExtrusionCrossSection=[1 1; -1 1; -1 -1; 1 -1]  ExtrusionCrossSectionUnits=m  ExtrusionLength=1  ExtrusionLengthUnits=m  PolygonNumSides=3  PolygonOuterRadius=1  PolygonOuterRadiusUnits=m  ExtGeomFileType=STEP  ExtGeomFileName=model/DYS-BLDC-86x10-BE8108-12-rotor_Default_sldprt.STEP  ExtGeomFileUnits=m  RevolutionCrossSection=[1 1; 1 -1; 2 -1; 2 1]  RevolutionCrossSectionUnits=m  RevolutionExtent=Full  RevolutionAngle=180  RevolutionAngleUnits=deg
  Transform : sm_lib/Frames and Transforms/Rigid Transform  TranslationMethod=Cartesian  TranslationStandardOffset=0  TranslationLengthUnit=mm  TranslationStandardAxis=+Z  TranslationCartesianOffset=minitaurParams.RigidTransform(20).translation  TranslationROffset=0  TranslationROffsetUnits=m  TranslationZOffset=0  TranslationZOffsetUnits=m  TranslationThetaOffset=0  TranslationThetaOffsetUnits=deg  RotationMethod=ArbitraryAxis  RotationAngleUnits=rad  RotationStandardAxis=+Z  RotationAngle=minitaurParams.RigidTransform(20).angle  RotationArbitraryAxis=minitaurParams.RigidTransform(20).axis  FollAlignAxisA=+X  BaseAlignAxisA=+Y  FollAlignAxisB=+Y  BaseAlignAxisB=+Z  RotationSequenceAxes=FollowerAxes  RotationSequence=XYX  RotationSequenceAngles=[0 0 0]  RotationSequenceAnglesUnits=deg  RotationMatrix=[1 0 0; 0 1 0; 0 0 1]
  Transform1 : sm_lib/Frames and Transforms/Rigid Transform  TranslationMethod=Cartesian  TranslationStandardOffset=0  TranslationLengthUnit=mm  TranslationStandardAxis=+Z  TranslationCartesianOffset=minitaurParams.RigidTransform(57).translation  TranslationROffset=0  TranslationROffsetUnits=m  TranslationZOffset=0  TranslationZOffsetUnits=m  TranslationThetaOffset=0  TranslationThetaOffsetUnits=deg  RotationMethod=ArbitraryAxis  RotationAngleUnits=rad  RotationStandardAxis=+Z  RotationAngle=minitaurParams.RigidTransform(57).angle  RotationArbitraryAxis=minitaurParams.RigidTransform(57).axis  FollAlignAxisA=+X  BaseAlignAxisA=+Y  FollAlignAxisB=+Y  BaseAlignAxisB=+Z  RotationSequenceAxes=FollowerAxes  RotationSequence=XYX  RotationSequenceAngles=[0 0 0]  RotationSequenceAnglesUnits=deg  RotationMatrix=[1 0 0; 0 1 0; 0 0 1]
  F1 : PMIOPort  Port=1  Side=Left
  F : PMIOPort  Port=2  Side=Left
  connections:
  ReferenceFrame/RConn1 -- Transform/LConn1 -- Transform1/LConn1 -- Solid/RConn1
  Transform/RConn1 -- F/RConn1
  Transform1/RConn1 -- F1/RConn1

== system simTopLevel/GR Minitaur/minitaur_motor_module_IIA/DYS_BLDC_86x10_BE8108_12/DYS_BLDC_86x10_BE8108_12_stator_1_RIGID ==
  ReferenceFrame : sm_lib/Frames and Transforms/Reference Frame
  Solid : sm_lib/Body Elements/Solid  InertiaType=Custom  Mass=minitaurParams.Solid(6).mass  MassUnits=kg  CenterOfMass=minitaurParams.Solid(6).CoM  CenterOfMassUnits=mm  MomentsOfInertia=minitaurParams.Solid(6).MoI  MomentsOfInertiaUnits=kg*mm^2  ProductsOfInertia=minitaurParams.Solid(6).PoI  ProductsOfInertiaUnits=kg*mm^2  DensityBased=on  Density=1000  DensityUnits=kg/(m^3)  DoExposeReferenceFrame=on  SerializedFrames=<Frames/>  GraphicType=FromGeometry  MarkerShape=Sphere  MarkerSize=10  GraphicVisPropType=SimpleVisualProperties  GraphicDiffuseColor=minitaurParams.Solid(6).color  GraphicSpecularColor=[0.5 0.5 0.5 1.0]  GraphicAmbientColor=[0.15 0.15 0.15 1.0]  GraphicEmissiveColor=[0.0 0.0 0.0 1.0]  GraphicShininess=75  GraphicOpacity=minitaurParams.Solid(6).opacity  GeometryShape=FromFile  RectangleSize=[1 1]  RectangleSizeUnits=m  BrickDimensions=[1 1 1]  BrickDimensionUnits=m  CylinderRadius=1  CylinderRadiusUnits=m  CylinderLength=1  CylinderLengthUnits=m  SphereRadius=1  SphereRadiusUnits=m  EllipsoidRadii=[1 1 1]  EllipsoidRadiiUnits=m  ExtrusionCrossSection=[1 1; -1 1; -1 -1; 1 -1]  ExtrusionCrossSectionUnits=m  ExtrusionLength=1  ExtrusionLengthUnits=m  PolygonNumSides=3  PolygonOuterRadius=1  PolygonOuterRadiusUnits=m  ExtGeomFileType=STEP  ExtGeomFileName=model/DYS-BLDC-86x10-BE8108-12-stator_Default_sldprt.STEP  ExtGeomFileUnits=m  RevolutionCrossSection=[1 1; 1 -1; 2 -1; 2 1]  RevolutionCrossSectionUnits=m  RevolutionExtent=Full  RevolutionAngle=180  RevolutionAngleUnits=deg
  Transform : sm_lib/Frames and Transforms/Rigid Transform  TranslationMethod=Cartesian  TranslationStandardOffset=0  TranslationLengthUnit=mm  TranslationStandardAxis=+Z  TranslationCartesianOffset=minitaurParams.RigidTransform(17).translation  TranslationROffset=0  TranslationROffsetUnits=m  TranslationZOffset=0  TranslationZOffsetUnits=m  TranslationThetaOffset=0  TranslationThetaOffsetUnits=deg  RotationMethod=ArbitraryAxis  RotationAngleUnits=rad  RotationStandardAxis=+Z  RotationAngle=minitaurParams.RigidTransform(17).angle  RotationArbitraryAxis=minitaurParams.RigidTransform(17).axis  FollAlignAxisA=+X  BaseAlignAxisA=+Y  FollAlignAxisB=+Y  BaseAlignAxisB=+Z  RotationSequenceAxes=FollowerAxes  RotationSequence=XYX  RotationSequenceAngles=[0 0 0]  RotationSequenceAnglesUnits=deg  RotationMatrix=[1 0 0; 0 1 0; 0 0 1]
  Transform1 : sm_lib/Frames and Transforms/Rigid Transform  TranslationMethod=Cartesian  TranslationStandardOffset=0  TranslationLengthUnit=mm  TranslationStandardAxis=+Z  TranslationCartesianOffset=minitaurParams.RigidTransform(19).translation  TranslationROffset=0  TranslationROffsetUnits=m  TranslationZOffset=0  TranslationZOffsetUnits=m  TranslationThetaOffset=0  TranslationThetaOffsetUnits=deg  RotationMethod=ArbitraryAxis  RotationAngleUnits=rad  RotationStandardAxis=+Z  RotationAngle=minitaurParams.RigidTransform(19).angle  RotationArbitraryAxis=minitaurParams.RigidTransform(19).axis  FollAlignAxisA=+X  BaseAlignAxisA=+Y  FollAlignAxisB=+Y  BaseAlignAxisB=+Z  RotationSequenceAxes=FollowerAxes  RotationSequence=XYX  RotationSequenceAngles=[0 0 0]  RotationSequenceAnglesUnits=deg  RotationMatrix=[1 0 0; 0 1 0; 0 0 1]
  Transform2 : sm_lib/Frames and Transforms/Rigid Transform  TranslationMethod=Cartesian  TranslationStandardOffset=0  TranslationLengthUnit=mm  TranslationStandardAxis=+Z  TranslationCartesianOffset=minitaurParams.RigidTransform(26).translation  TranslationROffset=0  TranslationROffsetUnits=m  TranslationZOffset=0  TranslationZOffsetUnits=m  TranslationThetaOffset=0  TranslationThetaOffsetUnits=deg  RotationMethod=ArbitraryAxis  RotationAngleUnits=rad  RotationStandardAxis=+Z  RotationAngle=minitaurParams.RigidTransform(26).angle  RotationArbitraryAxis=minitaurParams.RigidTransform(26).axis  FollAlignAxisA=+X  BaseAlignAxisA=+Y  FollAlignAxisB=+Y  BaseAlignAxisB=+Z  RotationSequenceAxes=FollowerAxes  RotationSequence=XYX  RotationSequenceAngles=[0 0 0]  RotationSequenceAnglesUnits=deg  RotationMatrix=[1 0 0; 0 1 0; 0 0 1]
  Transform3 : sm_lib/Frames and Transforms/Rigid Transform  TranslationMethod=Cartesian  TranslationStandardOffset=0  TranslationLengthUnit=mm  TranslationStandardAxis=+Z  TranslationCartesianOffset=minitaurParams.RigidTransform(32).translation  TranslationROffset=0  TranslationROffsetUnits=m  TranslationZOffset=0  TranslationZOffsetUnits=m  TranslationThetaOffset=0  TranslationThetaOffsetUnits=deg  RotationMethod=ArbitraryAxis  RotationAngleUnits=rad  RotationStandardAxis=+Z  RotationAngle=minitaurParams.RigidTransform(32).angle  RotationArbitraryAxis=minitaurParams.RigidTransform(32).axis  FollAlignAxisA=+X  BaseAlignAxisA=+Y  FollAlignAxisB=+Y  BaseAlignAxisB=+Z  RotationSequenceAxes=FollowerAxes  RotationSequence=XYX  RotationSequenceAngles=[0 0 0]  RotationSequenceAnglesUnits=deg  RotationMatrix=[1 0 0; 0 1 0; 0 0 1]
  F2 : PMIOPort  Port=1  Side=Left
  F3 : PMIOPort  Port=2  Side=Left
  F : PMIOPort  Port=3  Side=Left
  F1 : PMIOPort  Port=4  Side=Right
  connections:
  ReferenceFrame/RConn1 -- Solid/RConn1 -- Transform/LConn1 -- Transform1/LConn1 -- Transform2/LConn1 -- Transform3/LConn1
  Transform/RConn1 -- F/RConn1
  Transform1/RConn1 -- F1/RConn1
  Transform2/RConn1 -- F2/RConn1
  Transform3/RConn1 -- F3/RConn1

== system simTopLevel/GR Minitaur/minitaur_motor_module_IIB/DYS_BLDC_86x10_BE8108_12/BLDC Model ==
  Desired Torque  [Nm] : Inport
  Velocity [rad/s] : Inport  Port=2
  Constant : Constant  Value=torque_sat
  Constant1 : Constant  Value=-torque_sat
  Gain : Gain  Gain=1/kt
  Gain1 : Gain  Gain=r
  Math Function : Math  Operator=square  SaturateOnIntegerOverflow=on
  Saturation Dynamic : simulink/Discontinuities/Saturation Dynamic  OutMin=[]  OutMax=[]  OutDataTypeStr=Inherit: Same as second input  OutDataType=fixdt(1, 16)  OutScaling=2^-10  DoSatur=off
  Terminator : Terminator
  Transfer Fcn : TransferFcn  Denominator=[timeconst 1]
  Torque [N*m] : Outport
  Ploss [W] : Outport  Port=2
  wires:
  Desired Torque  [Nm]/1 -> Transfer Fcn/1
  Math Function/1 -> Gain1/1
  Gain/1 -> Math Function/1
  Gain1/1 -> Ploss [W]/1
  Velocity [rad/s]/1 -> Terminator/1
  Transfer Fcn/1 -> Saturation Dynamic/2
  Saturation Dynamic/1 -> Gain/1, Torque [N*m]/1
  Constant/1 -> Saturation Dynamic/1
  Constant1/1 -> Saturation Dynamic/3
